simulink model "VSD_FD_codegen_V2"  (R2021b)
settings: Solver=FixedStepDiscrete  StartTime=0.0  StopTime=2  RelTol=1e-3  EnableMultiTasking=on
PreLoadFcn:
  | uz_setCodegenPaths
model workspace (MATLAB code in the model file):
  | cmdLim = Simulink.Parameter;
  | cmdLim.Value = 15;
  | cmdLim.Description = 'Limit for controlling the maximum surface command angle.';
  | cmdLim.Min = 0;
  | cmdLim.Max = 90;
  | cmdLim.DocUnits = 'deg';
  | 
  | dispGain = Simulink.Parameter;
  | dispGain.Value = 0.75;
  | dispGain.Description = 'Gain applied to the displacement error.';
  | dispGain.Min = 0;
  | dispGain.Max = [];
  | dispGain.DocUnits = 'deg/sec/deg';
  | 
  | dispLim = Simulink.Parameter;
  | dispLim.Value = 30;
  | dispLim.Description = 'Limit for controlling the maximum commanded angle.';
  | dispLim.Min = 0;
  | dispLim.Max = 180;
  | dispLim.DocUnits = 'deg';
  | 
  | intGain = Simulink.Parameter;
  | intGain.Value = 0.5;
  | intGain.Description = 'Gain applied to the integral error.';
  | intGain.Min = 0;
  | intGain.Max = [];
  | intGain.DocUnits = 'deg/sec/deg/sec';
  | 
  | intLim = Simulink.Parameter;
  | intLim.Value = 5;
  | intLim.Description = 'Limit for controlling the maximum commanded angle.';
  | intLim.Min = 0;
  | intLim.Max = 90;
  | intLim.DocUnits = 'deg';
  | 
  | rateGain = Simulink.Parameter;
  | rateGain.Value = 2;
  | rateGain.Description = 'Gain applied to the rate error.';
  | rateGain.Min = 0;
  | rateGain.Max = [];
  | rateGain.DocUnits = 'deg/deg/sec';
  | 
  | rateLim = Simulink.Parameter;
  | rateLim.Value = 6;
  | rateLim.Description = 'Limit for controlling the maximum commanded angle.';
  | rateLim.Min = 0;
  | rateLim.Max = 180;
  | rateLim.DocUnits = 'deg/sec';
  | 
  | hdgGain = Simulink.Parameter;
  | hdgGain.Value = 0.015;
undefined symbols (not defined in the file or in its folder): DiscIntNeverNeededParam, f_FD
libraries: simulink x203, dspstat3 x3, spsFirstOrderFilterLib x2
(part 1 of 2)
settings Model: RequirementInfo={} %GIDa_fe9045fd_0412_4b6e_8206_617cc20e6fde  FPTRunName=Active  Creator=ts  LastModifiedBy=Josef Knoblach
settings SolverCC: AlgebraicLoopSolver=TrustRegion  PositivePriorityOrder=on  AutoInsertRateTranBlk=on
settings DataIOCC: SaveOutput=off  SignalLogging=off  DSMLogging=off  SaveTime=off
settings OptimizationCC: DefaultParameterBehavior=Inlined  UseDivisionForNetSlopeComputation=on  GainParamInheritBuiltInType=on  UseFloatMulNetSlope=on  UseSpecifiedMinMax=on  InlineInvariantSignals=on  PassReuseOutputArgsAs=Individual arguments  NoFixptDivByZeroProtection=on  EfficientFloat2IntCast=on  LifeSpan=1  MaxStackSize=64  OptimizeBlockOrder=speed  DifferentSizesBufferReuse=on  EfficientTunableParamExpr=on
settings DebuggingCC: AllowSymbolicDim=off  SFUnexpectedBacktrackingDiag=warning  SFNoUnconditionalDefaultTransitionDiag=warning  SFExecutionAtInitializationDiag=none  SFMachineParentedDataDiag=warning  ArithmeticOperatorsInVariantConditions=warning
settings HardwareCC: ProdBitPerPointer=32  ProdBitPerSizeT=32  ProdBitPerPtrDiffT=32  ProdLargestAtomicInteger=Long  ProdLargestAtomicFloat=Double  ProdWordSize=32  ProdLongLongMode=on  ProdHWDeviceType=ARM Compatible->ARM Cortex-R  HardwareBoardFeatureSet=SoCBlockset
settings SFSimCC: MATLABDynamicMemAlloc=off
settings RTWCC: Description=Embedded Coder  SystemTargetFile=ert.tlc  GenCodeOnly=on  TemplateMakefile=ert_default_tmf  GenerateReport=on  BuildConfiguration=Faster Runs  IncludeHyperlinkInReport=on  GenerateCodeMetricsReport=on  CheckMdlBeforeBuild=Warning
settings CodeAppCC: ForceParamTrailComments=on  IgnoreCustomStorageClasses=off  OperatorAnnotations=on  SimulinkDataObjDesc=on  SFDataObjDesc=on  MATLABFcnDesc=on  CustomSymbolStrGlobalVar=rt$N$M_$R  CustomSymbolStrType=$N$M_$R  CustomSymbolStrFcn=$N$M$F  CustomSymbolStrMacro=$N$M  InsertBlockDesc=on  StateflowObjectComments=on  MATLABSourceComments=on  EnableCustomComments=on  ReqsInCode=on
settings ERTTargetCC: TargetLangStandard=C99 (ISO)  CodeReplacementLibrary=GNU C99 extensions  MultiwordLength=2048  IncludeMdlTerminateFcn=off  CombineSignalStateStructs=on  SuppressErrorStatus=on  IncludeFileDelimiter=UseQuote  SupportAbsoluteTime=off  CodeInterfacePackaging=Reusable function  SupportNonFinite=off  RemoveResetFunc=off  InlinedParameterPlacement=NonHierarchical  MultiInstanceErrorCode=Warning  RootIOFormat=Part of model data structure  ERTCustomFileTemplate=example_file_process.tlc  GlobalDataDefinition=InSourceFile  GlobalDataReference=InSourceFile  ERTFilePackagingFormat=CompactWithDataFile
settings ConfigComp: CovScope=ReferencedModels  CovSaveName=covdata_rollAP  CovMetricSettings=dcmtrwe  CovHTMLOptions=-sRT=1 -aTS=1 -bRG=1 -bTC=1 -hTR=1 -nFC=0 -scm=1 -bcm=1 -xEv=0  CovSaveCumulativeToWorkspaceVar=on  CovSaveSingleToWorkspaceVar=on  CovCumulativeVarName=covCumulativeData_rollAP  CovReportOnPause=off  CovExternalEMLEnable=off  CovSFcnEnable=off

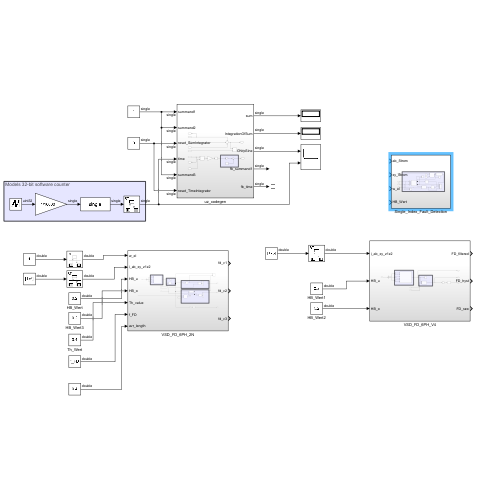
[thumbnail: Simulink's stored preview of the top-level diagram]
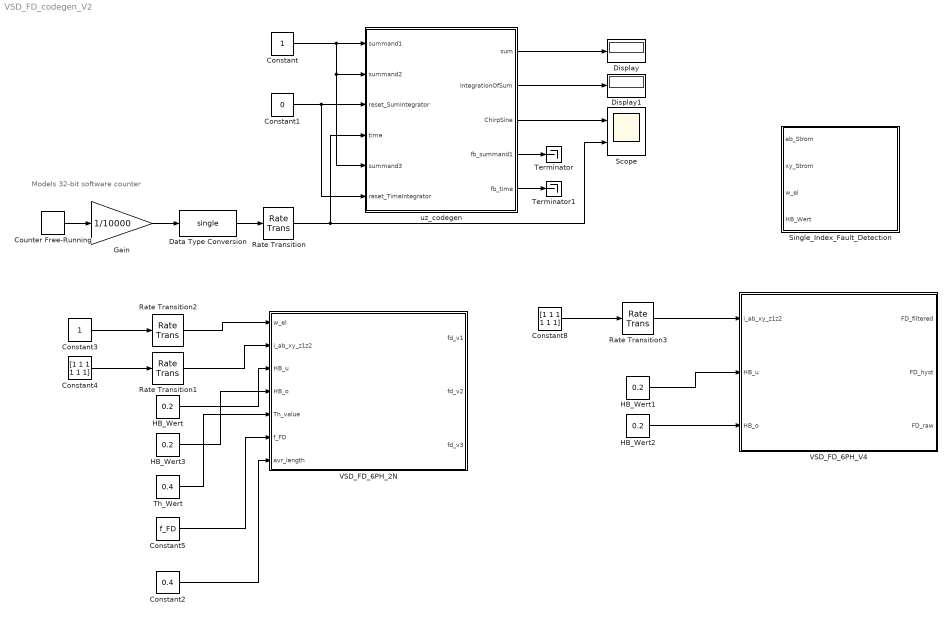
== system VSD_FD_codegen_V2 ==
  note: Models 32-bit software counter
  Constant : Constant  OutDataTypeStr=single  SampleTime=1/10000
  Constant1 : Constant  Value=0  OutDataTypeStr=single  SampleTime=1/10000
  Constant2 : Constant  Value=0.4
  Constant3 : Constant
  Constant4 : Constant  Value=[1 1 1 1 1 1]
  Constant5 : Constant  Value=f_FD
  Constant8 : Constant  Value=[1 1 1 1 1 1]
  Counter Free-Running : simulink/Sources/Counter Free-Running  NumBits=32  tsamp=1/10000
  Data Type Conversion : DataTypeConversion  OutDataTypeStr=single
  Display : Display
  Display1 : Display
  Gain : Gain  Gain=1/10000  OutDataTypeStr=single
  HB_Wert{,1..3} (4 alike) : Constant  Value=0.2
  Rate Transition : RateTransition  OutPortSampleTime=1/10000
  Rate Transition1 : RateTransition  OutPortSampleTime=1/f_FD
  Rate Transition2 : RateTransition  OutPortSampleTime=1/f_FD
  Rate Transition3 : RateTransition  OutPortSampleTime=1/f_FD
  Scope : Scope  NumInputPorts=2
  Single_Index_Fault_Detection : Subsystem
  Terminator : Terminator
  Terminator1 : Terminator
  Th_Wert : Constant  Value=0.4
  VSD_FD_6PH_2N : Subsystem
  VSD_FD_6PH_V4 : Subsystem
  uz_codegen : Subsystem
  wires:
  HB_Wert2/1 -> VSD_FD_6PH_V4/3(HB_o)
  HB_Wert/1 -> VSD_FD_6PH_2N/3(HB_u)
  Th_Wert/1 -> VSD_FD_6PH_2N/5(Th_value)
  Rate Transition1/1 -> VSD_FD_6PH_2N/2(i_ab_xy_z1z2)
  Constant5/1 -> VSD_FD_6PH_2N/6(f_FD)
  Rate Transition3/1 -> VSD_FD_6PH_V4/1(i_ab_xy_z1z2)
  Constant3/1 -> Rate Transition2/1
  Constant4/1 -> Rate Transition1/1
  Constant/1 -> uz_codegen/5(summand3), uz_codegen/2(summand2), uz_codegen/1(summand1)
  Constant1/1 -> uz_codegen/6(reset_TimeIntegrator), uz_codegen/3(reset_SumIntegrator)
  Gain/1 -> Data Type Conversion/1
  uz_codegen/5(fb_time) -> Terminator1/1
  Counter Free-Running/1 -> Gain/1
  HB_Wert3/1 -> VSD_FD_6PH_2N/4(HB_o)
  HB_Wert1/1 -> VSD_FD_6PH_V4/2(HB_u)
  uz_codegen/4(fb_summand1) -> Terminator/1
  Constant2/1 -> VSD_FD_6PH_2N/7(avr_length)
  Rate Transition/1 -> uz_codegen/4(time), Scope/2
  Data Type Conversion/1 -> Rate Transition/1
  Rate Transition2/1 -> VSD_FD_6PH_2N/1(w_el)
  uz_codegen/2(IntegrationOfSum) -> Display1/1
  uz_codegen/3(ChirpSine) -> Scope/1
  uz_codegen/1(sum) -> Display/1
  Constant8/1 -> Rate Transition3/1

== system VSD_FD_codegen_V2/Single_Index_Fault_Detection ==
  note: Single-Index-Methode
  ab_Strom : Inport
  xy_Strom : Inport  Port=2
  w_el : Inport  Port=3
  HB_Wert : Inport  Port=4
  Constant10 : Constant
  Constant11 : Constant  Value=f_FD
  Demux7 : Demux  Outputs=2
  Demux8 : Demux  Outputs=2
  HystereseBand1 : MATLAB Function  TreatAsAtomicUnit=on
  MATLAB Function2 : MATLAB Function  TreatAsAtomicUnit=on
  Moving Average1 : dspstat3/Moving Average  Method=Sliding window  ForgettingFactorPort=off  SpecifyWindowLength=on  WindowLength=50  ForgettingFactor=0.9  SimulateUsing=Code generation
  Moving Average3 : dspstat3/Moving Average  Method=Sliding window  ForgettingFactorPort=off  SpecifyWindowLength=on  WindowLength=25  ForgettingFactor=0.9  SimulateUsing=Code generation
  Scope16 : Scope  NumInputPorts=2
  Scope17 : Scope  NumInputPorts=2
  Scope2 : Scope  NumInputPorts=5
  Scope21 : Scope
  Single_Index : MATLAB Function  TreatAsAtomicUnit=on
  Subsystem5 : Subsystem
  wires:
  Demux8/1 -> Single_Index/3(i_x)
  HB_Wert/1 -> HystereseBand1/2(e)
  MATLAB Function2/1(N) -> Scope21/1, Subsystem5/2(Ordnung)
  Demux7/2 -> Single_Index/2(i_b)
  Single_Index/1(R) -> Subsystem5/1(x_n), Moving Average1/1, Scope2/1, HystereseBand1/1(Ri)
  HystereseBand1/1(Ro) -> Scope2/5, Moving Average3/1
  xy_Strom/1 -> Scope16/2, Demux8/1
  Moving Average1/1 -> Scope2/2
  Constant11/1 -> MATLAB Function2/2(f)
  Single_Index/2(A) -> Scope17/1
  Subsystem5/1(y_n) -> Scope2/4
  ab_Strom/1 -> Scope16/1, Demux7/1
  Demux7/1 -> Single_Index/1(i_a)
  Demux8/2 -> Single_Index/4(i_y)
  Single_Index/3(B) -> Scope17/2
  Moving Average3/1 -> Scope2/3
  Constant10/1 -> MATLAB Function2/3(k)
  w_el/1 -> MATLAB Function2/1(w_el)

== system VSD_FD_codegen_V2/VSD_FD_6PH_2N ==
  note: Hysterese
  note: 6-Index-VSD-FD
  note: Mittelwertbildung über Bruchteil einer Stromperiode mit FIR-Filter mit einstellbarer Länge (0-100)
  note: Mittelwertfilter Länge 50 als moving average Block + Auswertung
  w_el : Inport
  i_ab_xy_z1z2 : Inport  Port=2
  HB_u : Inport  Port=3
  HB_o : Inport  Port=4
  Th_value : Inport  Port=5
  f_FD : Inport  Port=6
  avr_length : Inport  Port=7
  Auswertung : MATLAB Function  TreatAsAtomicUnit=on
  Auswertung2 : MATLAB Function  TreatAsAtomicUnit=on
  Demux : Demux  Outputs=2
  Demux1 : Demux  Outputs=3
  Demux13 : Demux  Outputs=2
  Demux4 : Demux  Outputs=2
  Display : Display
  Display2 : Display
  Fehlerindexe_asym_6Ph_2N : MATLAB Function  TreatAsAtomicUnit=on
  First-Order Filter : spsFirstOrderFilterLib/First-Order Filter  FilterType=Lowpass  Tc=5e-3  Ts=1/5000  Initialize=off  Vac_Init=[0, 0, 60]  Vdc_Init=0  PlotResponse=off  FreqRange="[0,  200,  1]"
  HystereseBand : MATLAB Function  TreatAsAtomicUnit=on
  MATLAB Function1 : MATLAB Function  TreatAsAtomicUnit=on
  Moving Average2 : dspstat3/Moving Average  Method=Sliding window  ForgettingFactorPort=off  SpecifyWindowLength=on  WindowLength=30  ForgettingFactor=0.9  SimulateUsing=Code generation
  Reshape : Reshape  OutputDimensionality=Row vector (2-D)
  Reshape1 : Reshape  OutputDimensionality=Row vector (2-D)
  Scope13 : Scope  NumInputPorts=2
  Scope31 : Scope
  Scope7 : Scope  NumInputPorts=4
  Subsystem : Subsystem
  fd_v1 : Outport
  fd_v2 : Outport  Port=2
  fd_v3 : Outport  Port=3
  wires:
  Demux4/2 -> Fehlerindexe_asym_6Ph_2N/4(i_y)
  Auswertung/1(F) -> fd_v1/1, Display/1
  Demux/2 -> Fehlerindexe_asym_6Ph_2N/2(i_b)
  Moving Average2/1 -> Scope7/3, Auswertung/1(e)
  Demux/1 -> Fehlerindexe_asym_6Ph_2N/1(i_a)
  Auswertung2/1(F) -> fd_v2/1, Display2/1
  Fehlerindexe_asym_6Ph_2N/1(R) -> Scope31/1, HystereseBand/1(Ri)
  HB_u/1 -> HystereseBand/2(e_u)
  MATLAB Function1/1(N) -> Scope13/1, Subsystem/2(Ordnung)
  Demux4/1 -> Fehlerindexe_asym_6Ph_2N/3(i_x)
  HB_o/1 -> HystereseBand/3(e_o)
  Th_value/1 -> Auswertung/2(th), Auswertung2/2(th)
  Subsystem/1(y_n) -> Scope13/2, Auswertung2/1(e), Scope7/4
  Reshape/1 -> Moving Average2/1
  HystereseBand/1(Ro) -> Scope7/1, Reshape/1, Reshape1/1, Subsystem/1(x_n)
  Demux13/2 -> Fehlerindexe_asym_6Ph_2N/6(i_z2)
  Demux13/1 -> Fehlerindexe_asym_6Ph_2N/5(i_z1)
  Demux1/3 -> Demux13/1
  Demux1/2 -> Demux4/1
  Demux1/1 -> Demux/1
  w_el/1 -> MATLAB Function1/1(w_el)
  Reshape1/1 -> First-Order Filter/1
  i_ab_xy_z1z2/1 -> Demux1/1
  First-Order Filter/1 -> fd_v3/1
  f_FD/1 -> MATLAB Function1/2(f)
  avr_length/1 -> MATLAB Function1/3(k)

== system VSD_FD_codegen_V2/VSD_FD_6PH_V4 ==
  note: Hysterese
  note: 6-Index-VSD-FD
  i_ab_xy_z1z2 : Inport
  HB_u : Inport  Port=2
  HB_o : Inport  Port=3
  Demux : Demux  Outputs=2
  Demux1 : Demux  Outputs=3
  Demux13 : Demux  Outputs=2
  Demux4 : Demux  Outputs=2
  Fehlerindexe_asym_6Ph : MATLAB Function  TreatAsAtomicUnit=on
  First-Order Filter : spsFirstOrderFilterLib/First-Order Filter  FilterType=Lowpass  Tc=5e-3  Ts=1/f_FD  Initialize=off  Vac_Init=[0, 0, 60]  Vdc_Init=0  PlotResponse=off  FreqRange="[0,  200,  1]"
  HystereseBand : MATLAB Function  TreatAsAtomicUnit=on
  Reshape1 : Reshape  OutputDimensionality=Row vector (2-D)
  Scope31 : Scope
  FD_filtered : Outport
  FD_hyst : Outport  Port=2
  FD_raw : Outport  Port=3
  wires:
  Demux4/2 -> Fehlerindexe_asym_6Ph/4(i_y)
  Demux/2 -> Fehlerindexe_asym_6Ph/2(i_b)
  Demux/1 -> Fehlerindexe_asym_6Ph/1(i_a)
  Fehlerindexe_asym_6Ph/1(R) -> FD_raw/1, Scope31/1, HystereseBand/1(Ri)
  HB_u/1 -> HystereseBand/2(e_u)
  Demux4/1 -> Fehlerindexe_asym_6Ph/3(i_x)
  HB_o/1 -> HystereseBand/3(e_o)
  HystereseBand/1(Ro) -> FD_hyst/1, Reshape1/1
  Demux13/2 -> Fehlerindexe_asym_6Ph/6(i_z2)
  Demux13/1 -> Fehlerindexe_asym_6Ph/5(i_z1)
  Demux1/3 -> Demux13/1
  Demux1/2 -> Demux4/1
  Demux1/1 -> Demux/1
  Reshape1/1 -> First-Order Filter/1
  i_ab_xy_z1z2/1 -> Demux1/1
  First-Order Filter/1 -> FD_filtered/1

== system VSD_FD_codegen_V2/uz_codegen ==
  note: Offset sine to 0..1 for PWM module
  summand1 : Inport  OutDataTypeStr=single
  summand2 : Inport  Port=2  OutDataTypeStr=single
  reset_SumIntegrator : Inport  Port=3  OutDataTypeStr=single
  time : Inport  Port=4  OutDataTypeStr=single
  summand3 : Inport  Port=5  OutDataTypeStr=single
  reset_TimeIntegrator : Inport  Port=6  OutDataTypeStr=single
  Constant : Constant  Value=0.5  OutDataTypeStr=single
  Discrete-Time Integrator : DiscreteIntegrator  ExternalReset=level  SampleTime=-1  UpperSaturationLimit=1000  LowerSaturationLimit=-1000  ICPrevOutput=DiscIntNeverNeededParam  ICPrevScaledInput=DiscIntNeverNeededParam
  Discrete-Time Integrator2 : DiscreteIntegrator  ExternalReset=level  SampleTime=-1  UpperSaturationLimit=1000  LowerSaturationLimit=-1000  ICPrevOutput=DiscIntNeverNeededParam  ICPrevScaledInput=DiscIntNeverNeededParam
  Gain1 : Gain  Gain=2*pi
  Gain2 : Gain  Gain=0.5
  Sum : Sum  Inputs=+++  InputSameDT=on  OutDataTypeStr=Inherit: Same as first input
  Sum3 : Sum  Inputs=|++
  Trigonometric Function : Trigonometry
  sum : Outport  VectorParamsAs1DForOutWhenUnconnected=off
  IntegrationOfSum : Outport  Port=2  VectorParamsAs1DForOutWhenUnconnected=off
  ChirpSine : Outport  Port=3  VectorParamsAs1DForOutWhenUnconnected=off
  fb_summand1 : Outport  Port=4  VectorParamsAs1DForOutWhenUnconnected=off
  fb_time : Outport  Port=5  VectorParamsAs1DForOutWhenUnconnected=off
  wires:
  summand1/1 -> Sum/1, fb_summand1/1
  summand2/1 -> Sum/2
  Sum/1 -> sum/1, Discrete-Time Integrator/1
  Discrete-Time Integrator/1 -> IntegrationOfSum/1
  Gain1/1 -> Trigonometric Function/1
  Trigonometric Function/1 -> Gain2/1
  Gain2/1 -> Sum3/1
  Constant/1 -> Sum3/2
  Sum3/1 -> ChirpSine/1
  time/1 -> fb_time/1, Discrete-Time Integrator2/1
  reset_SumIntegrator/1 -> Discrete-Time Integrator/2
  Discrete-Time Integrator2/1 -> Gain1/1
  summand3/1 -> Sum/3
  reset_TimeIntegrator/1 -> Discrete-Time Integrator2/2

== system VSD_FD_codegen_V2/Single_Index_Fault_Detection/Subsystem5 ==
  note: Erinnerung: Filterordnung ist 1 kleiner als die FIlter Länge
      | Filter-Ordnung = Anzahl Delays
      | Als Eingangswert wird die Ordnung verwendet, zu diese
  x_n : Inport
  Ordnung : Inport  Port=2
  Compare To Constant : simulink/Logic and Bit Operations/Compare To Constant  relop=>=  const=0  OutDataTypeStr=boolean
  Constant : Constant  Value=-1
  Constant1 : Constant
  Divide : Product  Inputs=*/
  Element_10_O : Subsystem
      settings: PortSchema="{\"entries\":[{\"content\":{\"sides\":[{\"content\":{\"connectorIds\":[\"In1\",\"In2\",\"In3\",\"Out4\"]},\"type\":\"ConnectorPlacement.EquallySpacedRectSide\",\"uuid\":\"2b5c73c0-de94-4d49-9ce4-b0167bdc4750\"},{\"content\":{\"connectorIds\":[\"Out1\",\"Out2\",\"Out3\",\"In4\"],\"side\":\"RIGHT\"},\"type\":\"ConnectorPlacement.EquallySpacedRectSide\",\"uuid\":\"96b282bd-6b41-4201-930f-ecc5f93ba408\"},{\"content\":{\"connectorIds\":[],\"side\":\"TOP\"},\"type\":\"ConnectorPlacement.EquallySpacedRectSide\",\"uuid\":\"027867ac-4e73-422f-a0ae-a587b47092bb\"}]},\"type\":\"ConnectorPlacement.EquallySpacedConnector\",\"uuid\":\"c6f63bf1-14c9-4725-bc9e-a23fbf01be21\"}],\"packageUris\":[\"http://schema.mathworks.com/mf0/Connector/R2020b\"],\"version\":\"1.0\"}"
  Element_10_O1 : Subsystem
      settings: PortSchema="{\"entries\":[{\"content\":{\"sides\":[{\"content\":{\"connectorIds\":[\"In1\",\"In2\",\"In3\",\"Out4\"]},\"type\":\"ConnectorPlacement.EquallySpacedRectSide\",\"uuid\":\"2b5c73c0-de94-4d49-9ce4-b0167bdc4750\"},{\"content\":{\"connectorIds\":[\"Out1\",\"Out2\",\"Out3\",\"In4\"],\"side\":\"RIGHT\"},\"type\":\"ConnectorPlacement.EquallySpacedRectSide\",\"uuid\":\"96b282bd-6b41-4201-930f-ecc5f93ba408\"},{\"content\":{\"connectorIds\":[],\"side\":\"TOP\"},\"type\":\"ConnectorPlacement.EquallySpacedRectSide\",\"uuid\":\"027867ac-4e73-422f-a0ae-a587b47092bb\"}]},\"type\":\"ConnectorPlacement.EquallySpacedConnector\",\"uuid\":\"c6f63bf1-14c9-4725-bc9e-a23fbf01be21\"}],\"packageUris\":[\"http://schema.mathworks.com/mf0/Connector/R2020b\"],\"version\":\"1.0\"}"
  Element_10_O2 : Subsystem
      settings: PortSchema="{\"entries\":[{\"content\":{\"sides\":[{\"content\":{\"connectorIds\":[\"In1\",\"In2\",\"In3\",\"Out4\"]},\"type\":\"ConnectorPlacement.EquallySpacedRectSide\",\"uuid\":\"2b5c73c0-de94-4d49-9ce4-b0167bdc4750\"},{\"content\":{\"connectorIds\":[\"Out1\",\"Out2\",\"Out3\",\"In4\"],\"side\":\"RIGHT\"},\"type\":\"ConnectorPlacement.EquallySpacedRectSide\",\"uuid\":\"96b282bd-6b41-4201-930f-ecc5f93ba408\"},{\"content\":{\"connectorIds\":[],\"side\":\"TOP\"},\"type\":\"ConnectorPlacement.EquallySpacedRectSide\",\"uuid\":\"027867ac-4e73-422f-a0ae-a587b47092bb\"}]},\"type\":\"ConnectorPlacement.EquallySpacedConnector\",\"uuid\":\"c6f63bf1-14c9-4725-bc9e-a23fbf01be21\"}],\"packageUris\":[\"http://schema.mathworks.com/mf0/Connector/R2020b\"],\"version\":\"1.0\"}"
  Element_10_O3 : Subsystem
      settings: PortSchema="{\"entries\":[{\"content\":{\"sides\":[{\"content\":{\"connectorIds\":[\"In1\",\"In2\",\"In3\",\"Out4\"]},\"type\":\"ConnectorPlacement.EquallySpacedRectSide\",\"uuid\":\"2b5c73c0-de94-4d49-9ce4-b0167bdc4750\"},{\"content\":{\"connectorIds\":[\"Out1\",\"Out2\",\"Out3\",\"In4\"],\"side\":\"RIGHT\"},\"type\":\"ConnectorPlacement.EquallySpacedRectSide\",\"uuid\":\"96b282bd-6b41-4201-930f-ecc5f93ba408\"},{\"content\":{\"connectorIds\":[],\"side\":\"TOP\"},\"type\":\"ConnectorPlacement.EquallySpacedRectSide\",\"uuid\":\"027867ac-4e73-422f-a0ae-a587b47092bb\"}]},\"type\":\"ConnectorPlacement.EquallySpacedConnector\",\"uuid\":\"c6f63bf1-14c9-4725-bc9e-a23fbf01be21\"}],\"packageUris\":[\"http://schema.mathworks.com/mf0/Connector/R2020b\"],\"version\":\"1.0\"}"
  Element_10_O4 : Subsystem
      settings: PortSchema="{\"entries\":[{\"content\":{\"sides\":[{\"content\":{\"connectorIds\":[\"In1\",\"In2\",\"In3\",\"Out4\"]},\"type\":\"ConnectorPlacement.EquallySpacedRectSide\",\"uuid\":\"2b5c73c0-de94-4d49-9ce4-b0167bdc4750\"},{\"content\":{\"connectorIds\":[\"Out1\",\"Out2\",\"Out3\",\"In4\"],\"side\":\"RIGHT\"},\"type\":\"ConnectorPlacement.EquallySpacedRectSide\",\"uuid\":\"96b282bd-6b41-4201-930f-ecc5f93ba408\"},{\"content\":{\"connectorIds\":[],\"side\":\"TOP\"},\"type\":\"ConnectorPlacement.EquallySpacedRectSide\",\"uuid\":\"027867ac-4e73-422f-a0ae-a587b47092bb\"}]},\"type\":\"ConnectorPlacement.EquallySpacedConnector\",\"uuid\":\"c6f63bf1-14c9-4725-bc9e-a23fbf01be21\"}],\"packageUris\":[\"http://schema.mathworks.com/mf0/Connector/R2020b\"],\"version\":\"1.0\"}"
  Element_10_O5 : Subsystem
      settings: PortSchema="{\"entries\":[{\"content\":{\"sides\":[{\"content\":{\"connectorIds\":[\"In1\",\"In2\",\"In3\",\"Out4\"]},\"type\":\"ConnectorPlacement.EquallySpacedRectSide\",\"uuid\":\"2b5c73c0-de94-4d49-9ce4-b0167bdc4750\"},{\"content\":{\"connectorIds\":[\"Out1\",\"Out2\",\"Out3\",\"In4\"],\"side\":\"RIGHT\"},\"type\":\"ConnectorPlacement.EquallySpacedRectSide\",\"uuid\":\"96b282bd-6b41-4201-930f-ecc5f93ba408\"},{\"content\":{\"connectorIds\":[],\"side\":\"TOP\"},\"type\":\"ConnectorPlacement.EquallySpacedRectSide\",\"uuid\":\"027867ac-4e73-422f-a0ae-a587b47092bb\"}]},\"type\":\"ConnectorPlacement.EquallySpacedConnector\",\"uuid\":\"c6f63bf1-14c9-4725-bc9e-a23fbf01be21\"}],\"packageUris\":[\"http://schema.mathworks.com/mf0/Connector/R2020b\"],\"version\":\"1.0\"}"
  Element_10_O6 : Subsystem
      settings: PortSchema="{\"entries\":[{\"content\":{\"sides\":[{\"content\":{\"connectorIds\":[\"In1\",\"In2\",\"In3\",\"Out4\"]},\"type\":\"ConnectorPlacement.EquallySpacedRectSide\",\"uuid\":\"2b5c73c0-de94-4d49-9ce4-b0167bdc4750\"},{\"content\":{\"connectorIds\":[\"Out1\",\"Out2\",\"Out3\",\"In4\"],\"side\":\"RIGHT\"},\"type\":\"ConnectorPlacement.EquallySpacedRectSide\",\"uuid\":\"96b282bd-6b41-4201-930f-ecc5f93ba408\"},{\"content\":{\"connectorIds\":[],\"side\":\"TOP\"},\"type\":\"ConnectorPlacement.EquallySpacedRectSide\",\"uuid\":\"027867ac-4e73-422f-a0ae-a587b47092bb\"}]},\"type\":\"ConnectorPlacement.EquallySpacedConnector\",\"uuid\":\"c6f63bf1-14c9-4725-bc9e-a23fbf01be21\"}],\"packageUris\":[\"http://schema.mathworks.com/mf0/Connector/R2020b\"],\"version\":\"1.0\"}"
  Element_10_O7 : Subsystem
      settings: PortSchema="{\"entries\":[{\"content\":{\"sides\":[{\"content\":{\"connectorIds\":[\"In1\",\"In2\",\"In3\",\"Out4\"]},\"type\":\"ConnectorPlacement.EquallySpacedRectSide\",\"uuid\":\"2b5c73c0-de94-4d49-9ce4-b0167bdc4750\"},{\"content\":{\"connectorIds\":[\"Out1\",\"Out2\",\"Out3\",\"In4\"],\"side\":\"RIGHT\"},\"type\":\"ConnectorPlacement.EquallySpacedRectSide\",\"uuid\":\"96b282bd-6b41-4201-930f-ecc5f93ba408\"},{\"content\":{\"connectorIds\":[],\"side\":\"TOP\"},\"type\":\"ConnectorPlacement.EquallySpacedRectSide\",\"uuid\":\"027867ac-4e73-422f-a0ae-a587b47092bb\"}]},\"type\":\"ConnectorPlacement.EquallySpacedConnector\",\"uuid\":\"c6f63bf1-14c9-4725-bc9e-a23fbf01be21\"}],\"packageUris\":[\"http://schema.mathworks.com/mf0/Connector/R2020b\"],\"version\":\"1.0\"}"
  Element_10_O8 : Subsystem
      settings: PortSchema="{\"entries\":[{\"content\":{\"sides\":[{\"content\":{\"connectorIds\":[\"In1\",\"In2\",\"In3\",\"Out4\"]},\"type\":\"ConnectorPlacement.EquallySpacedRectSide\",\"uuid\":\"2b5c73c0-de94-4d49-9ce4-b0167bdc4750\"},{\"content\":{\"connectorIds\":[\"Out1\",\"Out2\",\"Out3\",\"In4\"],\"side\":\"RIGHT\"},\"type\":\"ConnectorPlacement.EquallySpacedRectSide\",\"uuid\":\"96b282bd-6b41-4201-930f-ecc5f93ba408\"},{\"content\":{\"connectorIds\":[],\"side\":\"TOP\"},\"type\":\"ConnectorPlacement.EquallySpacedRectSide\",\"uuid\":\"027867ac-4e73-422f-a0ae-a587b47092bb\"}]},\"type\":\"ConnectorPlacement.EquallySpacedConnector\",\"uuid\":\"c6f63bf1-14c9-4725-bc9e-a23fbf01be21\"}],\"packageUris\":[\"http://schema.mathworks.com/mf0/Connector/R2020b\"],\"version\":\"1.0\"}"
  Element_10_O9 : Subsystem
      settings: PortSchema="{\"entries\":[{\"content\":{\"sides\":[{\"content\":{\"connectorIds\":[\"In1\",\"In2\",\"In3\",\"Out4\"]},\"type\":\"ConnectorPlacement.EquallySpacedRectSide\",\"uuid\":\"2b5c73c0-de94-4d49-9ce4-b0167bdc4750\"},{\"content\":{\"connectorIds\":[\"Out1\",\"Out2\",\"Out3\",\"In4\"],\"side\":\"RIGHT\"},\"type\":\"ConnectorPlacement.EquallySpacedRectSide\",\"uuid\":\"96b282bd-6b41-4201-930f-ecc5f93ba408\"},{\"content\":{\"connectorIds\":[],\"side\":\"TOP\"},\"type\":\"ConnectorPlacement.EquallySpacedRectSide\",\"uuid\":\"027867ac-4e73-422f-a0ae-a587b47092bb\"}]},\"type\":\"ConnectorPlacement.EquallySpacedConnector\",\"uuid\":\"c6f63bf1-14c9-4725-bc9e-a23fbf01be21\"}],\"packageUris\":[\"http://schema.mathworks.com/mf0/Connector/R2020b\"],\"version\":\"1.0\"}"
  Product1 : Product
  Sum : Sum  Inputs=++|
  Sum129 : Sum  Inputs=++|
  y_n : Outport
  wires:
  x_n/1 -> Product1/2, Element_10_O/3(x_i)
  Compare To Constant/1 -> Product1/1
  Product1/1 -> Sum/1
  Constant/1 -> Element_10_O/1(in_1)
  Sum/1 -> Divide/1
  Divide/1 -> y_n/1
  Sum129/1 -> Divide/2
  Constant1/1 -> Sum129/1
  Ordnung/1 -> Element_10_O/2(L_i), Compare To Constant/1, Sum129/2
  Element_10_O/4(y_o) -> Sum/2
  Element_10_O/1(out_1) -> Element_10_O1/1(in_1)
  Element_10_O/2(L_o) -> Element_10_O1/2(L_i)
  Element_10_O/3(x_o) -> Element_10_O1/3(x_i)
  Element_10_O1/4(y_o) -> Element_10_O/4(y_i)
  Element_10_O3/1(out_1) -> Element_10_O4/1(in_1)
  Element_10_O3/2(L_o) -> Element_10_O4/2(L_i)
  Element_10_O3/3(x_o) -> Element_10_O4/3(x_i)
  Element_10_O4/4(y_o) -> Element_10_O3/4(y_i)
  Element_10_O2/1(out_1) -> Element_10_O3/1(in_1)
  Element_10_O2/2(L_o) -> Element_10_O3/2(L_i)
  Element_10_O2/3(x_o) -> Element_10_O3/3(x_i)
  Element_10_O3/4(y_o) -> Element_10_O2/4(y_i)
  Element_10_O1/1(out_1) -> Element_10_O2/1(in_1)
  Element_10_O1/2(L_o) -> Element_10_O2/2(L_i)
  Element_10_O1/3(x_o) -> Element_10_O2/3(x_i)
  Element_10_O2/4(y_o) -> Element_10_O1/4(y_i)
  Element_10_O8/2(L_o) -> Element_10_O9/2(L_i)
  Element_10_O8/3(x_o) -> Element_10_O9/3(x_i)
  Element_10_O7/2(L_o) -> Element_10_O8/2(L_i)
  Element_10_O9/4(y_o) -> Element_10_O8/4(y_i)
  Element_10_O7/3(x_o) -> Element_10_O8/3(x_i)
  Element_10_O8/1(out_1) -> Element_10_O9/1(in_1)
  Element_10_O6/1(out_1) -> Element_10_O7/1(in_1)
  Element_10_O7/4(y_o) -> Element_10_O6/4(y_i)
  Element_10_O8/4(y_o) -> Element_10_O7/4(y_i)
  Element_10_O6/4(y_o) -> Element_10_O5/4(y_i)
  Element_10_O7/1(out_1) -> Element_10_O8/1(in_1)
  Element_10_O6/3(x_o) -> Element_10_O7/3(x_i)
  Element_10_O5/3(x_o) -> Element_10_O6/3(x_i)
  Element_10_O6/2(L_o) -> Element_10_O7/2(L_i)
  Element_10_O5/2(L_o) -> Element_10_O6/2(L_i)
  Element_10_O5/1(out_1) -> Element_10_O6/1(in_1)
  Element_10_O4/1(out_1) -> Element_10_O5/1(in_1)
  Element_10_O4/2(L_o) -> Element_10_O5/2(L_i)
  Element_10_O4/3(x_o) -> Element_10_O5/3(x_i)
  Element_10_O5/4(y_o) -> Element_10_O4/4(y_i)

== system VSD_FD_codegen_V2/VSD_FD_6PH_2N/Subsystem ==
  note: Erinnerung: Filterordnung ist 1 kleiner als die FIlter Länge
      | Filter-Ordnung = Anzahl Delays
      | Als Eingangswert wird die Ordnung verwendet, zu diese
  x_n : Inport
  Ordnung : Inport  Port=2
  Compare To Constant : simulink/Logic and Bit Operations/Compare To Constant  relop=>=  const=0  OutDataTypeStr=boolean
  Constant : Constant  Value=-1
  Constant1 : Constant
  Divide : Product  Inputs=*/
  Element_10_O : Subsystem
      settings: PortSchema="{\"entries\":[{\"content\":{\"sides\":[{\"content\":{\"connectorIds\":[\"In1\",\"In2\",\"In3\",\"Out4\"]},\"type\":\"ConnectorPlacement.EquallySpacedRectSide\",\"uuid\":\"2b5c73c0-de94-4d49-9ce4-b0167bdc4750\"},{\"content\":{\"connectorIds\":[\"Out1\",\"Out2\",\"Out3\",\"In4\"],\"side\":\"RIGHT\"},\"type\":\"ConnectorPlacement.EquallySpacedRectSide\",\"uuid\":\"96b282bd-6b41-4201-930f-ecc5f93ba408\"},{\"content\":{\"connectorIds\":[],\"side\":\"TOP\"},\"type\":\"ConnectorPlacement.EquallySpacedRectSide\",\"uuid\":\"027867ac-4e73-422f-a0ae-a587b47092bb\"}]},\"type\":\"ConnectorPlacement.EquallySpacedConnector\",\"uuid\":\"c6f63bf1-14c9-4725-bc9e-a23fbf01be21\"}],\"packageUris\":[\"http://schema.mathworks.com/mf0/Connector/R2020b\"],\"version\":\"1.0\"}"
  Element_10_O1 : Subsystem
      settings: PortSchema="{\"entries\":[{\"content\":{\"sides\":[{\"content\":{\"connectorIds\":[\"In1\",\"In2\",\"In3\",\"Out4\"]},\"type\":\"ConnectorPlacement.EquallySpacedRectSide\",\"uuid\":\"2b5c73c0-de94-4d49-9ce4-b0167bdc4750\"},{\"content\":{\"connectorIds\":[\"Out1\",\"Out2\",\"Out3\",\"In4\"],\"side\":\"RIGHT\"},\"type\":\"ConnectorPlacement.EquallySpacedRectSide\",\"uuid\":\"96b282bd-6b41-4201-930f-ecc5f93ba408\"},{\"content\":{\"connectorIds\":[],\"side\":\"TOP\"},\"type\":\"ConnectorPlacement.EquallySpacedRectSide\",\"uuid\":\"027867ac-4e73-422f-a0ae-a587b47092bb\"}]},\"type\":\"ConnectorPlacement.EquallySpacedConnector\",\"uuid\":\"c6f63bf1-14c9-4725-bc9e-a23fbf01be21\"}],\"packageUris\":[\"http://schema.mathworks.com/mf0/Connector/R2020b\"],\"version\":\"1.0\"}"
  Element_10_O2 : Subsystem
      settings: PortSchema="{\"entries\":[{\"content\":{\"sides\":[{\"content\":{\"connectorIds\":[\"In1\",\"In2\",\"In3\",\"Out4\"]},\"type\":\"ConnectorPlacement.EquallySpacedRectSide\",\"uuid\":\"2b5c73c0-de94-4d49-9ce4-b0167bdc4750\"},{\"content\":{\"connectorIds\":[\"Out1\",\"Out2\",\"Out3\",\"In4\"],\"side\":\"RIGHT\"},\"type\":\"ConnectorPlacement.EquallySpacedRectSide\",\"uuid\":\"96b282bd-6b41-4201-930f-ecc5f93ba408\"},{\"content\":{\"connectorIds\":[],\"side\":\"TOP\"},\"type\":\"ConnectorPlacement.EquallySpacedRectSide\",\"uuid\":\"027867ac-4e73-422f-a0ae-a587b47092bb\"}]},\"type\":\"ConnectorPlacement.EquallySpacedConnector\",\"uuid\":\"c6f63bf1-14c9-4725-bc9e-a23fbf01be21\"}],\"packageUris\":[\"http://schema.mathworks.com/mf0/Connector/R2020b\"],\"version\":\"1.0\"}"
  Element_10_O3 : Subsystem
      settings: PortSchema="{\"entries\":[{\"content\":{\"sides\":[{\"content\":{\"connectorIds\":[\"In1\",\"In2\",\"In3\",\"Out4\"]},\"type\":\"ConnectorPlacement.EquallySpacedRectSide\",\"uuid\":\"2b5c73c0-de94-4d49-9ce4-b0167bdc4750\"},{\"content\":{\"connectorIds\":[\"Out1\",\"Out2\",\"Out3\",\"In4\"],\"side\":\"RIGHT\"},\"type\":\"ConnectorPlacement.EquallySpacedRectSide\",\"uuid\":\"96b282bd-6b41-4201-930f-ecc5f93ba408\"},{\"content\":{\"connectorIds\":[],\"side\":\"TOP\"},\"type\":\"ConnectorPlacement.EquallySpacedRectSide\",\"uuid\":\"027867ac-4e73-422f-a0ae-a587b47092bb\"}]},\"type\":\"ConnectorPlacement.EquallySpacedConnector\",\"uuid\":\"c6f63bf1-14c9-4725-bc9e-a23fbf01be21\"}],\"packageUris\":[\"http://schema.mathworks.com/mf0/Connector/R2020b\"],\"version\":\"1.0\"}"
  Element_10_O4 : Subsystem
      settings: PortSchema="{\"entries\":[{\"content\":{\"sides\":[{\"content\":{\"connectorIds\":[\"In1\",\"In2\",\"In3\",\"Out4\"]},\"type\":\"ConnectorPlacement.EquallySpacedRectSide\",\"uuid\":\"2b5c73c0-de94-4d49-9ce4-b0167bdc4750\"},{\"content\":{\"connectorIds\":[\"Out1\",\"Out2\",\"Out3\",\"In4\"],\"side\":\"RIGHT\"},\"type\":\"ConnectorPlacement.EquallySpacedRectSide\",\"uuid\":\"96b282bd-6b41-4201-930f-ecc5f93ba408\"},{\"content\":{\"connectorIds\":[],\"side\":\"TOP\"},\"type\":\"ConnectorPlacement.EquallySpacedRectSide\",\"uuid\":\"027867ac-4e73-422f-a0ae-a587b47092bb\"}]},\"type\":\"ConnectorPlacement.EquallySpacedConnector\",\"uuid\":\"c6f63bf1-14c9-4725-bc9e-a23fbf01be21\"}],\"packageUris\":[\"http://schema.mathworks.com/mf0/Connector/R2020b\"],\"version\":\"1.0\"}"
  Element_10_O5 : Subsystem
      settings: PortSchema="{\"entries\":[{\"content\":{\"sides\":[{\"content\":{\"connectorIds\":[\"In1\",\"In2\",\"In3\",\"Out4\"]},\"type\":\"ConnectorPlacement.EquallySpacedRectSide\",\"uuid\":\"2b5c73c0-de94-4d49-9ce4-b0167bdc4750\"},{\"content\":{\"connectorIds\":[\"Out1\",\"Out2\",\"Out3\",\"In4\"],\"side\":\"RIGHT\"},\"type\":\"ConnectorPlacement.EquallySpacedRectSide\",\"uuid\":\"96b282bd-6b41-4201-930f-ecc5f93ba408\"},{\"content\":{\"connectorIds\":[],\"side\":\"TOP\"},\"type\":\"ConnectorPlacement.EquallySpacedRectSide\",\"uuid\":\"027867ac-4e73-422f-a0ae-a587b47092bb\"}]},\"type\":\"ConnectorPlacement.EquallySpacedConnector\",\"uuid\":\"c6f63bf1-14c9-4725-bc9e-a23fbf01be21\"}],\"packageUris\":[\"http://schema.mathworks.com/mf0/Connector/R2020b\"],\"version\":\"1.0\"}"
  Element_10_O6 : Subsystem
      settings: PortSchema="{\"entries\":[{\"content\":{\"sides\":[{\"content\":{\"connectorIds\":[\"In1\",\"In2\",\"In3\",\"Out4\"]},\"type\":\"ConnectorPlacement.EquallySpacedRectSide\",\"uuid\":\"2b5c73c0-de94-4d49-9ce4-b0167bdc4750\"},{\"content\":{\"connectorIds\":[\"Out1\",\"Out2\",\"Out3\",\"In4\"],\"side\":\"RIGHT\"},\"type\":\"ConnectorPlacement.EquallySpacedRectSide\",\"uuid\":\"96b282bd-6b41-4201-930f-ecc5f93ba408\"},{\"content\":{\"connectorIds\":[],\"side\":\"TOP\"},\"type\":\"ConnectorPlacement.EquallySpacedRectSide\",\"uuid\":\"027867ac-4e73-422f-a0ae-a587b47092bb\"}]},\"type\":\"ConnectorPlacement.EquallySpacedConnector\",\"uuid\":\"c6f63bf1-14c9-4725-bc9e-a23fbf01be21\"}],\"packageUris\":[\"http://schema.mathworks.com/mf0/Connector/R2020b\"],\"version\":\"1.0\"}"
  Element_10_O7 : Subsystem
      settings: PortSchema="{\"entries\":[{\"content\":{\"sides\":[{\"content\":{\"connectorIds\":[\"In1\",\"In2\",\"In3\",\"Out4\"]},\"type\":\"ConnectorPlacement.EquallySpacedRectSide\",\"uuid\":\"2b5c73c0-de94-4d49-9ce4-b0167bdc4750\"},{\"content\":{\"connectorIds\":[\"Out1\",\"Out2\",\"Out3\",\"In4\"],\"side\":\"RIGHT\"},\"type\":\"ConnectorPlacement.EquallySpacedRectSide\",\"uuid\":\"96b282bd-6b41-4201-930f-ecc5f93ba408\"},{\"content\":{\"connectorIds\":[],\"side\":\"TOP\"},\"type\":\"ConnectorPlacement.EquallySpacedRectSide\",\"uuid\":\"027867ac-4e73-422f-a0ae-a587b47092bb\"}]},\"type\":\"ConnectorPlacement.EquallySpacedConnector\",\"uuid\":\"c6f63bf1-14c9-4725-bc9e-a23fbf01be21\"}],\"packageUris\":[\"http://schema.mathworks.com/mf0/Connector/R2020b\"],\"version\":\"1.0\"}"
  Element_10_O8 : Subsystem
      settings: PortSchema="{\"entries\":[{\"content\":{\"sides\":[{\"content\":{\"connectorIds\":[\"In1\",\"In2\",\"In3\",\"Out4\"]},\"type\":\"ConnectorPlacement.EquallySpacedRectSide\",\"uuid\":\"2b5c73c0-de94-4d49-9ce4-b0167bdc4750\"},{\"content\":{\"connectorIds\":[\"Out1\",\"Out2\",\"Out3\",\"In4\"],\"side\":\"RIGHT\"},\"type\":\"ConnectorPlacement.EquallySpacedRectSide\",\"uuid\":\"96b282bd-6b41-4201-930f-ecc5f93ba408\"},{\"content\":{\"connectorIds\":[],\"side\":\"TOP\"},\"type\":\"ConnectorPlacement.EquallySpacedRectSide\",\"uuid\":\"027867ac-4e73-422f-a0ae-a587b47092bb\"}]},\"type\":\"ConnectorPlacement.EquallySpacedConnector\",\"uuid\":\"c6f63bf1-14c9-4725-bc9e-a23fbf01be21\"}],\"packageUris\":[\"http://schema.mathworks.com/mf0/Connector/R2020b\"],\"version\":\"1.0\"}"
  Element_10_O9 : Subsystem
      settings: PortSchema="{\"entries\":[{\"content\":{\"sides\":[{\"content\":{\"connectorIds\":[\"In1\",\"In2\",\"In3\",\"Out4\"]},\"type\":\"ConnectorPlacement.EquallySpacedRectSide\",\"uuid\":\"2b5c73c0-de94-4d49-9ce4-b0167bdc4750\"},{\"content\":{\"connectorIds\":[\"Out1\",\"Out2\",\"Out3\",\"In4\"],\"side\":\"RIGHT\"},\"type\":\"ConnectorPlacement.EquallySpacedRectSide\",\"uuid\":\"96b282bd-6b41-4201-930f-ecc5f93ba408\"},{\"content\":{\"connectorIds\":[],\"side\":\"TOP\"},\"type\":\"ConnectorPlacement.EquallySpacedRectSide\",\"uuid\":\"027867ac-4e73-422f-a0ae-a587b47092bb\"}]},\"type\":\"ConnectorPlacement.EquallySpacedConnector\",\"uuid\":\"c6f63bf1-14c9-4725-bc9e-a23fbf01be21\"}],\"packageUris\":[\"http://schema.mathworks.com/mf0/Connector/R2020b\"],\"version\":\"1.0\"}"
  Product1 : Product
  Sum : Sum  Inputs=++|
  Sum129 : Sum  Inputs=++|
  y_n : Outport
  wires:
  x_n/1 -> Product1/2, Element_10_O/3(x_i)
  Compare To Constant/1 -> Product1/1
  Product1/1 -> Sum/1
  Constant/1 -> Element_10_O/1(in_1)
  Sum/1 -> Divide/1
  Divide/1 -> y_n/1
  Sum129/1 -> Divide/2
  Constant1/1 -> Sum129/1
  Ordnung/1 -> Element_10_O/2(L_i), Compare To Constant/1, Sum129/2
  Element_10_O/4(y_o) -> Sum/2
  Element_10_O/1(out_1) -> Element_10_O1/1(in_1)
  Element_10_O/2(L_o) -> Element_10_O1/2(L_i)
  Element_10_O/3(x_o) -> Element_10_O1/3(x_i)
  Element_10_O1/4(y_o) -> Element_10_O/4(y_i)
  Element_10_O3/1(out_1) -> Element_10_O4/1(in_1)
  Element_10_O3/2(L_o) -> Element_10_O4/2(L_i)
  Element_10_O3/3(x_o) -> Element_10_O4/3(x_i)
  Element_10_O4/4(y_o) -> Element_10_O3/4(y_i)
  Element_10_O2/1(out_1) -> Element_10_O3/1(in_1)
  Element_10_O2/2(L_o) -> Element_10_O3/2(L_i)
  Element_10_O2/3(x_o) -> Element_10_O3/3(x_i)
  Element_10_O3/4(y_o) -> Element_10_O2/4(y_i)
  Element_10_O1/1(out_1) -> Element_10_O2/1(in_1)
  Element_10_O1/2(L_o) -> Element_10_O2/2(L_i)
  Element_10_O1/3(x_o) -> Element_10_O2/3(x_i)
  Element_10_O2/4(y_o) -> Element_10_O1/4(y_i)
  Element_10_O8/2(L_o) -> Element_10_O9/2(L_i)
  Element_10_O8/3(x_o) -> Element_10_O9/3(x_i)
  Element_10_O7/2(L_o) -> Element_10_O8/2(L_i)
  Element_10_O9/4(y_o) -> Element_10_O8/4(y_i)
  Element_10_O7/3(x_o) -> Element_10_O8/3(x_i)
  Element_10_O8/1(out_1) -> Element_10_O9/1(in_1)
  Element_10_O6/1(out_1) -> Element_10_O7/1(in_1)
  Element_10_O7/4(y_o) -> Element_10_O6/4(y_i)
  Element_10_O8/4(y_o) -> Element_10_O7/4(y_i)
  Element_10_O6/4(y_o) -> Element_10_O5/4(y_i)
  Element_10_O7/1(out_1) -> Element_10_O8/1(in_1)
  Element_10_O6/3(x_o) -> Element_10_O7/3(x_i)
  Element_10_O5/3(x_o) -> Element_10_O6/3(x_i)
  Element_10_O6/2(L_o) -> Element_10_O7/2(L_i)
  Element_10_O5/2(L_o) -> Element_10_O6/2(L_i)
  Element_10_O5/1(out_1) -> Element_10_O6/1(in_1)
  Element_10_O4/1(out_1) -> Element_10_O5/1(in_1)
  Element_10_O4/2(L_o) -> Element_10_O5/2(L_i)
  Element_10_O4/3(x_o) -> Element_10_O5/3(x_i)
  Element_10_O5/4(y_o) -> Element_10_O4/4(y_i)

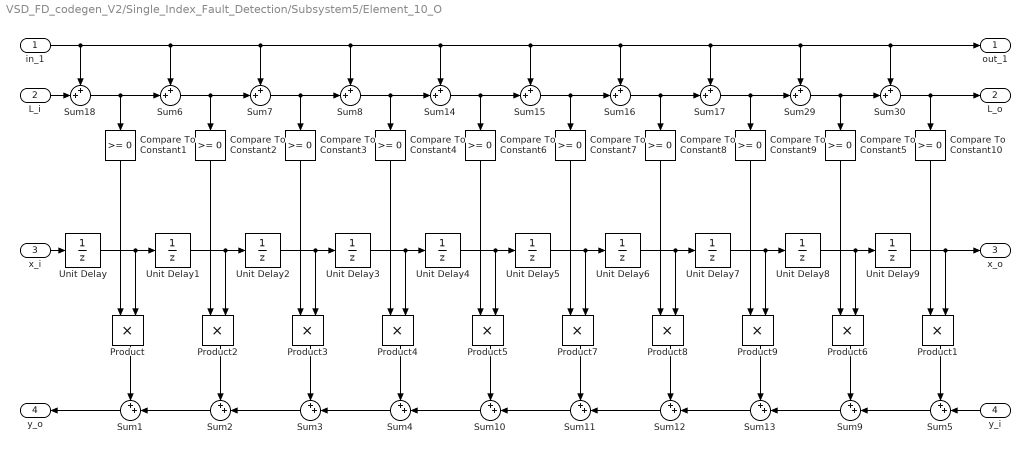
== system VSD_FD_codegen_V2/Single_Index_Fault_Detection/Subsystem5/Element_10_O ==
  in_1 : Inport
  L_i : Inport  Port=2
  x_i : Inport  Port=3
  y_i : Inport  Port=4
  Compare To Constant{1..10} (10 alike) : simulink/Logic and Bit Operations/Compare To Constant  relop=>=  const=0  OutDataTypeStr=boolean
  Product{,1..9} (10 alike) : Product
  Sum{1..18,29..30} (20 alike) : Sum  Inputs=++|
  Unit Delay{,1..9} (10 alike) : UnitDelay  SampleTime=-1  HasFrameUpgradeWarning=on
  out_1 : Outport
  L_o : Outport  Port=2
  x_o : Outport  Port=3
  y_o : Outport  Port=4
  wires:
  Sum2/1 -> Sum1/2
  Unit Delay4/1 -> Unit Delay5/1, Product5/2
  Unit Delay9/1 -> x_o/1, Product1/2
  Sum3/1 -> Sum2/2
  Sum6/1 -> Compare To Constant2/1, Sum7/2
  Sum15/1 -> Compare To Constant7/1, Sum16/2
  Sum9/1 -> Sum13/2
  Sum14/1 -> Sum15/2, Compare To Constant6/1
  Compare To Constant4/1 -> Product4/1
  Unit Delay7/1 -> Unit Delay8/1, Product9/2
  Unit Delay6/1 -> Unit Delay7/1, Product8/2
  Sum7/1 -> Compare To Constant3/1, Sum8/2
  Compare To Constant3/1 -> Product3/1
  Product8/1 -> Sum12/1
  Sum13/1 -> Sum12/2
  in_1/1 -> Sum18/1, Sum6/1, Sum7/1, Sum15/1, Sum16/1, out_1/1, Sum30/1, Sum29/1, Sum17/1, Sum14/1, Sum8/1
  Unit Delay8/1 -> Unit Delay9/1, Product6/2
  Product9/1 -> Sum13/1
  Sum11/1 -> Sum10/2
  Sum8/1 -> Compare To Constant4/1, Sum14/2
  Compare To Constant6/1 -> Product5/1
  Product7/1 -> Sum11/1
  Compare To Constant8/1 -> Product8/1
  Product/1 -> Sum1/1
  Unit Delay5/1 -> Unit Delay6/1, Product7/2
  Unit Delay/1 -> Unit Delay1/1, Product/2
  Unit Delay1/1 -> Unit Delay2/1, Product2/2
  Compare To Constant5/1 -> Product6/1
  Sum10/1 -> Sum4/2
  Sum1/1 -> y_o/1
  Compare To Constant2/1 -> Product2/1
  Sum16/1 -> Compare To Constant8/1, Sum17/2
  Compare To Constant1/1 -> Product/1
  Sum4/1 -> Sum3/2
  Sum17/1 -> Sum29/2, Compare To Constant9/1
  Unit Delay3/1 -> Unit Delay4/1, Product4/2
  Product5/1 -> Sum10/1
  Product6/1 -> Sum9/1
  Sum12/1 -> Sum11/2
  Sum29/1 -> Sum30/2, Compare To Constant5/1
  Sum30/1 -> L_o/1, Compare To Constant10/1
  Product4/1 -> Sum4/1
  Product2/1 -> Sum2/1
  Unit Delay2/1 -> Unit Delay3/1, Product3/2
  Compare To Constant9/1 -> Product9/1
  Product3/1 -> Sum3/1
  x_i/1 -> Unit Delay/1
  Compare To Constant7/1 -> Product7/1
  Compare To Constant10/1 -> Product1/1
  Product1/1 -> Sum5/1
  y_i/1 -> Sum5/2
  Sum5/1 -> Sum9/2
  L_i/1 -> Sum18/2
  Sum18/1 -> Compare To Constant1/1, Sum6/2

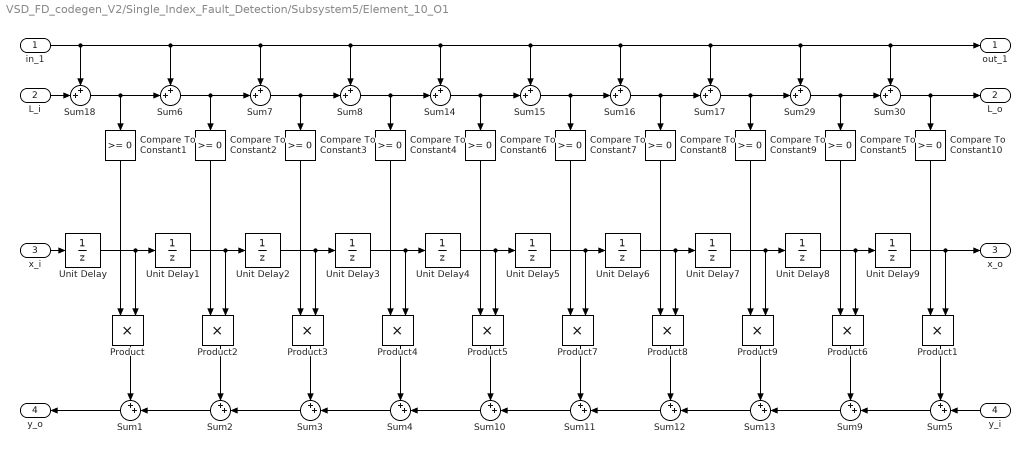
== system VSD_FD_codegen_V2/Single_Index_Fault_Detection/Subsystem5/Element_10_O1 ==
  in_1 : Inport
  L_i : Inport  Port=2
  x_i : Inport  Port=3
  y_i : Inport  Port=4
  Compare To Constant{1..10} (10 alike) : simulink/Logic and Bit Operations/Compare To Constant  relop=>=  const=0  OutDataTypeStr=boolean
  Product{,1..9} (10 alike) : Product
  Sum{1..18,29..30} (20 alike) : Sum  Inputs=++|
  Unit Delay{,1..9} (10 alike) : UnitDelay  SampleTime=-1  HasFrameUpgradeWarning=on
  out_1 : Outport
  L_o : Outport  Port=2
  x_o : Outport  Port=3
  y_o : Outport  Port=4
  wires:
  Sum2/1 -> Sum1/2
  Unit Delay4/1 -> Unit Delay5/1, Product5/2
  Unit Delay9/1 -> x_o/1, Product1/2
  Sum3/1 -> Sum2/2
  Sum6/1 -> Compare To Constant2/1, Sum7/2
  Sum15/1 -> Compare To Constant7/1, Sum16/2
  Sum9/1 -> Sum13/2
  Sum14/1 -> Sum15/2, Compare To Constant6/1
  Compare To Constant4/1 -> Product4/1
  Unit Delay7/1 -> Unit Delay8/1, Product9/2
  Unit Delay6/1 -> Unit Delay7/1, Product8/2
  Sum7/1 -> Compare To Constant3/1, Sum8/2
  Compare To Constant3/1 -> Product3/1
  Product8/1 -> Sum12/1
  Sum13/1 -> Sum12/2
  in_1/1 -> Sum18/1, Sum6/1, Sum7/1, Sum15/1, Sum16/1, out_1/1, Sum30/1, Sum29/1, Sum17/1, Sum14/1, Sum8/1
  Unit Delay8/1 -> Unit Delay9/1, Product6/2
  Product9/1 -> Sum13/1
  Sum11/1 -> Sum10/2
  Sum8/1 -> Compare To Constant4/1, Sum14/2
  Compare To Constant6/1 -> Product5/1
  Product7/1 -> Sum11/1
  Compare To Constant8/1 -> Product8/1
  Product/1 -> Sum1/1
  Unit Delay5/1 -> Unit Delay6/1, Product7/2
  Unit Delay/1 -> Unit Delay1/1, Product/2
  Unit Delay1/1 -> Unit Delay2/1, Product2/2
  Compare To Constant5/1 -> Product6/1
  Sum10/1 -> Sum4/2
  Sum1/1 -> y_o/1
  Compare To Constant2/1 -> Product2/1
  Sum16/1 -> Compare To Constant8/1, Sum17/2
  Compare To Constant1/1 -> Product/1
  Sum4/1 -> Sum3/2
  Sum17/1 -> Sum29/2, Compare To Constant9/1
  Unit Delay3/1 -> Unit Delay4/1, Product4/2
  Product5/1 -> Sum10/1
  Product6/1 -> Sum9/1
  Sum12/1 -> Sum11/2
  Sum29/1 -> Sum30/2, Compare To Constant5/1
  Sum30/1 -> L_o/1, Compare To Constant10/1
  Product4/1 -> Sum4/1
  Product2/1 -> Sum2/1
  Unit Delay2/1 -> Unit Delay3/1, Product3/2
  Compare To Constant9/1 -> Product9/1
  Product3/1 -> Sum3/1
  x_i/1 -> Unit Delay/1
  Compare To Constant7/1 -> Product7/1
  Compare To Constant10/1 -> Product1/1
  Product1/1 -> Sum5/1
  y_i/1 -> Sum5/2
  Sum5/1 -> Sum9/2
  L_i/1 -> Sum18/2
  Sum18/1 -> Compare To Constant1/1, Sum6/2

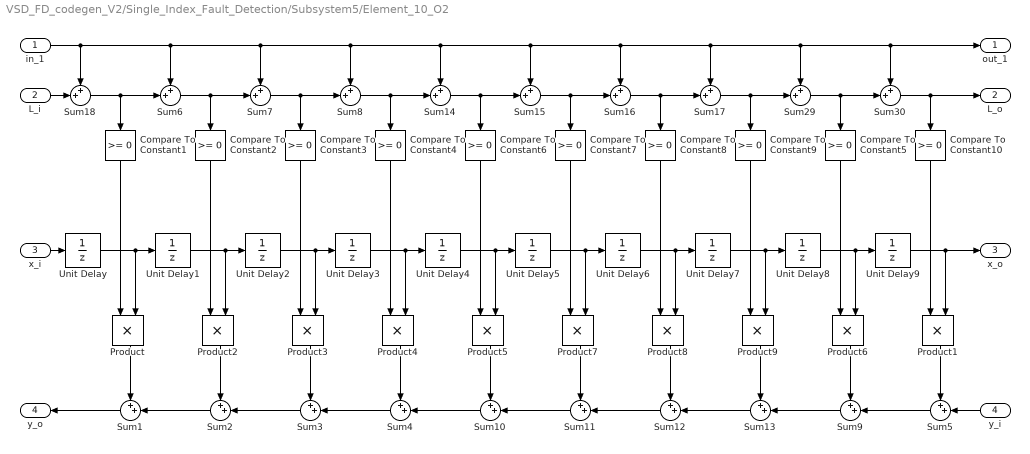
== system VSD_FD_codegen_V2/Single_Index_Fault_Detection/Subsystem5/Element_10_O2 ==
  in_1 : Inport
  L_i : Inport  Port=2
  x_i : Inport  Port=3
  y_i : Inport  Port=4
  Compare To Constant{1..10} (10 alike) : simulink/Logic and Bit Operations/Compare To Constant  relop=>=  const=0  OutDataTypeStr=boolean
  Product{,1..9} (10 alike) : Product
  Sum{1..18,29..30} (20 alike) : Sum  Inputs=++|
  Unit Delay{,1..9} (10 alike) : UnitDelay  SampleTime=-1  HasFrameUpgradeWarning=on
  out_1 : Outport
  L_o : Outport  Port=2
  x_o : Outport  Port=3
  y_o : Outport  Port=4
  wires:
  Sum2/1 -> Sum1/2
  Unit Delay4/1 -> Unit Delay5/1, Product5/2
  Unit Delay9/1 -> x_o/1, Product1/2
  Sum3/1 -> Sum2/2
  Sum6/1 -> Compare To Constant2/1, Sum7/2
  Sum15/1 -> Compare To Constant7/1, Sum16/2
  Sum9/1 -> Sum13/2
  Sum14/1 -> Sum15/2, Compare To Constant6/1
  Compare To Constant4/1 -> Product4/1
  Unit Delay7/1 -> Unit Delay8/1, Product9/2
  Unit Delay6/1 -> Unit Delay7/1, Product8/2
  Sum7/1 -> Compare To Constant3/1, Sum8/2
  Compare To Constant3/1 -> Product3/1
  Product8/1 -> Sum12/1
  Sum13/1 -> Sum12/2
  in_1/1 -> Sum18/1, Sum6/1, Sum7/1, Sum15/1, Sum16/1, out_1/1, Sum30/1, Sum29/1, Sum17/1, Sum14/1, Sum8/1
  Unit Delay8/1 -> Unit Delay9/1, Product6/2
  Product9/1 -> Sum13/1
  Sum11/1 -> Sum10/2
  Sum8/1 -> Compare To Constant4/1, Sum14/2
  Compare To Constant6/1 -> Product5/1
  Product7/1 -> Sum11/1
  Compare To Constant8/1 -> Product8/1
  Product/1 -> Sum1/1
  Unit Delay5/1 -> Unit Delay6/1, Product7/2
  Unit Delay/1 -> Unit Delay1/1, Product/2
  Unit Delay1/1 -> Unit Delay2/1, Product2/2
  Compare To Constant5/1 -> Product6/1
  Sum10/1 -> Sum4/2
  Sum1/1 -> y_o/1
  Compare To Constant2/1 -> Product2/1
  Sum16/1 -> Compare To Constant8/1, Sum17/2
  Compare To Constant1/1 -> Product/1
  Sum4/1 -> Sum3/2
  Sum17/1 -> Sum29/2, Compare To Constant9/1
  Unit Delay3/1 -> Unit Delay4/1, Product4/2
  Product5/1 -> Sum10/1
  Product6/1 -> Sum9/1
  Sum12/1 -> Sum11/2
  Sum29/1 -> Sum30/2, Compare To Constant5/1
  Sum30/1 -> L_o/1, Compare To Constant10/1
  Product4/1 -> Sum4/1
  Product2/1 -> Sum2/1
  Unit Delay2/1 -> Unit Delay3/1, Product3/2
  Compare To Constant9/1 -> Product9/1
  Product3/1 -> Sum3/1
  x_i/1 -> Unit Delay/1
  Compare To Constant7/1 -> Product7/1
  Compare To Constant10/1 -> Product1/1
  Product1/1 -> Sum5/1
  y_i/1 -> Sum5/2
  Sum5/1 -> Sum9/2
  L_i/1 -> Sum18/2
  Sum18/1 -> Compare To Constant1/1, Sum6/2

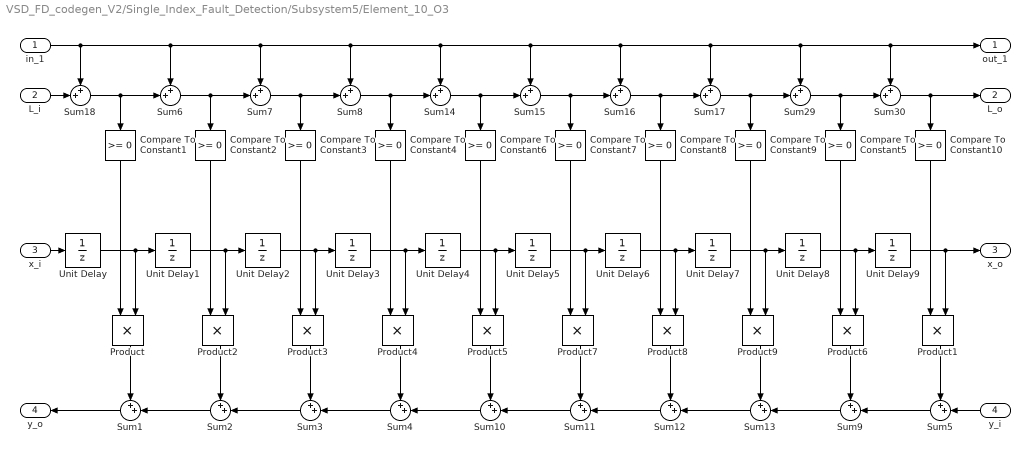
== system VSD_FD_codegen_V2/Single_Index_Fault_Detection/Subsystem5/Element_10_O3 ==
  in_1 : Inport
  L_i : Inport  Port=2
  x_i : Inport  Port=3
  y_i : Inport  Port=4
  Compare To Constant{1..10} (10 alike) : simulink/Logic and Bit Operations/Compare To Constant  relop=>=  const=0  OutDataTypeStr=boolean
  Product{,1..9} (10 alike) : Product
  Sum{1..18,29..30} (20 alike) : Sum  Inputs=++|
  Unit Delay{,1..9} (10 alike) : UnitDelay  SampleTime=-1  HasFrameUpgradeWarning=on
  out_1 : Outport
  L_o : Outport  Port=2
  x_o : Outport  Port=3
  y_o : Outport  Port=4
  wires:
  Sum2/1 -> Sum1/2
  Unit Delay4/1 -> Unit Delay5/1, Product5/2
  Unit Delay9/1 -> x_o/1, Product1/2
  Sum3/1 -> Sum2/2
  Sum6/1 -> Compare To Constant2/1, Sum7/2
  Sum15/1 -> Compare To Constant7/1, Sum16/2
  Sum9/1 -> Sum13/2
  Sum14/1 -> Sum15/2, Compare To Constant6/1
  Compare To Constant4/1 -> Product4/1
  Unit Delay7/1 -> Unit Delay8/1, Product9/2
  Unit Delay6/1 -> Unit Delay7/1, Product8/2
  Sum7/1 -> Compare To Constant3/1, Sum8/2
  Compare To Constant3/1 -> Product3/1
  Product8/1 -> Sum12/1
  Sum13/1 -> Sum12/2
  in_1/1 -> Sum18/1, Sum6/1, Sum7/1, Sum15/1, Sum16/1, out_1/1, Sum30/1, Sum29/1, Sum17/1, Sum14/1, Sum8/1
  Unit Delay8/1 -> Unit Delay9/1, Product6/2
  Product9/1 -> Sum13/1
  Sum11/1 -> Sum10/2
  Sum8/1 -> Compare To Constant4/1, Sum14/2
  Compare To Constant6/1 -> Product5/1
  Product7/1 -> Sum11/1
  Compare To Constant8/1 -> Product8/1
  Product/1 -> Sum1/1
  Unit Delay5/1 -> Unit Delay6/1, Product7/2
  Unit Delay/1 -> Unit Delay1/1, Product/2
  Unit Delay1/1 -> Unit Delay2/1, Product2/2
  Compare To Constant5/1 -> Product6/1
  Sum10/1 -> Sum4/2
  Sum1/1 -> y_o/1
  Compare To Constant2/1 -> Product2/1
  Sum16/1 -> Compare To Constant8/1, Sum17/2
  Compare To Constant1/1 -> Product/1
  Sum4/1 -> Sum3/2
  Sum17/1 -> Sum29/2, Compare To Constant9/1
  Unit Delay3/1 -> Unit Delay4/1, Product4/2
  Product5/1 -> Sum10/1
  Product6/1 -> Sum9/1
  Sum12/1 -> Sum11/2
  Sum29/1 -> Sum30/2, Compare To Constant5/1
  Sum30/1 -> L_o/1, Compare To Constant10/1
  Product4/1 -> Sum4/1
  Product2/1 -> Sum2/1
  Unit Delay2/1 -> Unit Delay3/1, Product3/2
  Compare To Constant9/1 -> Product9/1
  Product3/1 -> Sum3/1
  x_i/1 -> Unit Delay/1
  Compare To Constant7/1 -> Product7/1
  Compare To Constant10/1 -> Product1/1
  Product1/1 -> Sum5/1
  y_i/1 -> Sum5/2
  Sum5/1 -> Sum9/2
  L_i/1 -> Sum18/2
  Sum18/1 -> Compare To Constant1/1, Sum6/2

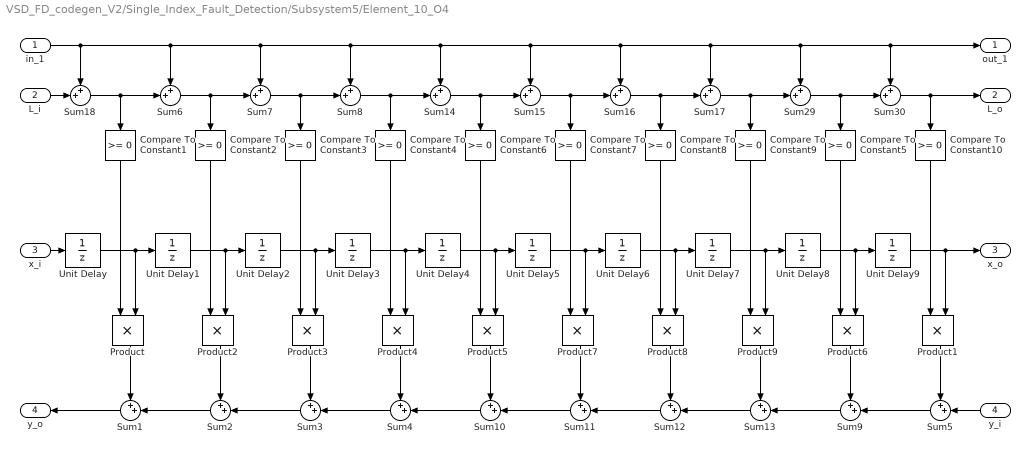
== system VSD_FD_codegen_V2/Single_Index_Fault_Detection/Subsystem5/Element_10_O4 ==
  in_1 : Inport
  L_i : Inport  Port=2
  x_i : Inport  Port=3
  y_i : Inport  Port=4
  Compare To Constant{1..10} (10 alike) : simulink/Logic and Bit Operations/Compare To Constant  relop=>=  const=0  OutDataTypeStr=boolean
  Product{,1..9} (10 alike) : Product
  Sum{1..18,29..30} (20 alike) : Sum  Inputs=++|
  Unit Delay{,1..9} (10 alike) : UnitDelay  SampleTime=-1  HasFrameUpgradeWarning=on
  out_1 : Outport
  L_o : Outport  Port=2
  x_o : Outport  Port=3
  y_o : Outport  Port=4
  wires:
  Sum2/1 -> Sum1/2
  Unit Delay4/1 -> Unit Delay5/1, Product5/2
  Unit Delay9/1 -> x_o/1, Product1/2
  Sum3/1 -> Sum2/2
  Sum6/1 -> Compare To Constant2/1, Sum7/2
  Sum15/1 -> Compare To Constant7/1, Sum16/2
  Sum9/1 -> Sum13/2
  Sum14/1 -> Sum15/2, Compare To Constant6/1
  Compare To Constant4/1 -> Product4/1
  Unit Delay7/1 -> Unit Delay8/1, Product9/2
  Unit Delay6/1 -> Unit Delay7/1, Product8/2
  Sum7/1 -> Compare To Constant3/1, Sum8/2
  Compare To Constant3/1 -> Product3/1
  Product8/1 -> Sum12/1
  Sum13/1 -> Sum12/2
  in_1/1 -> Sum18/1, Sum6/1, Sum7/1, Sum15/1, Sum16/1, out_1/1, Sum30/1, Sum29/1, Sum17/1, Sum14/1, Sum8/1
  Unit Delay8/1 -> Unit Delay9/1, Product6/2
  Product9/1 -> Sum13/1
  Sum11/1 -> Sum10/2
  Sum8/1 -> Compare To Constant4/1, Sum14/2
  Compare To Constant6/1 -> Product5/1
  Product7/1 -> Sum11/1
  Compare To Constant8/1 -> Product8/1
  Product/1 -> Sum1/1
  Unit Delay5/1 -> Unit Delay6/1, Product7/2
  Unit Delay/1 -> Unit Delay1/1, Product/2
  Unit Delay1/1 -> Unit Delay2/1, Product2/2
  Compare To Constant5/1 -> Product6/1
  Sum10/1 -> Sum4/2
  Sum1/1 -> y_o/1
  Compare To Constant2/1 -> Product2/1
  Sum16/1 -> Compare To Constant8/1, Sum17/2
  Compare To Constant1/1 -> Product/1
  Sum4/1 -> Sum3/2
  Sum17/1 -> Sum29/2, Compare To Constant9/1
  Unit Delay3/1 -> Unit Delay4/1, Product4/2
  Product5/1 -> Sum10/1
  Product6/1 -> Sum9/1
  Sum12/1 -> Sum11/2
  Sum29/1 -> Sum30/2, Compare To Constant5/1
  Sum30/1 -> L_o/1, Compare To Constant10/1
  Product4/1 -> Sum4/1
  Product2/1 -> Sum2/1
  Unit Delay2/1 -> Unit Delay3/1, Product3/2
  Compare To Constant9/1 -> Product9/1
  Product3/1 -> Sum3/1
  x_i/1 -> Unit Delay/1
  Compare To Constant7/1 -> Product7/1
  Compare To Constant10/1 -> Product1/1
  Product1/1 -> Sum5/1
  y_i/1 -> Sum5/2
  Sum5/1 -> Sum9/2
  L_i/1 -> Sum18/2
  Sum18/1 -> Compare To Constant1/1, Sum6/2
